simulink model "windModel"  (R2021a)
settings: Solver=VariableStepAuto  StartTime=0.0  StopTime=inf  RelTol=1e-3
undefined symbols (not defined in the file or in its folder): aircraft, FandM, MAV, plotprob
libraries: simulink x4
settings Model: Creator=DELL  LastModifiedBy=DELL

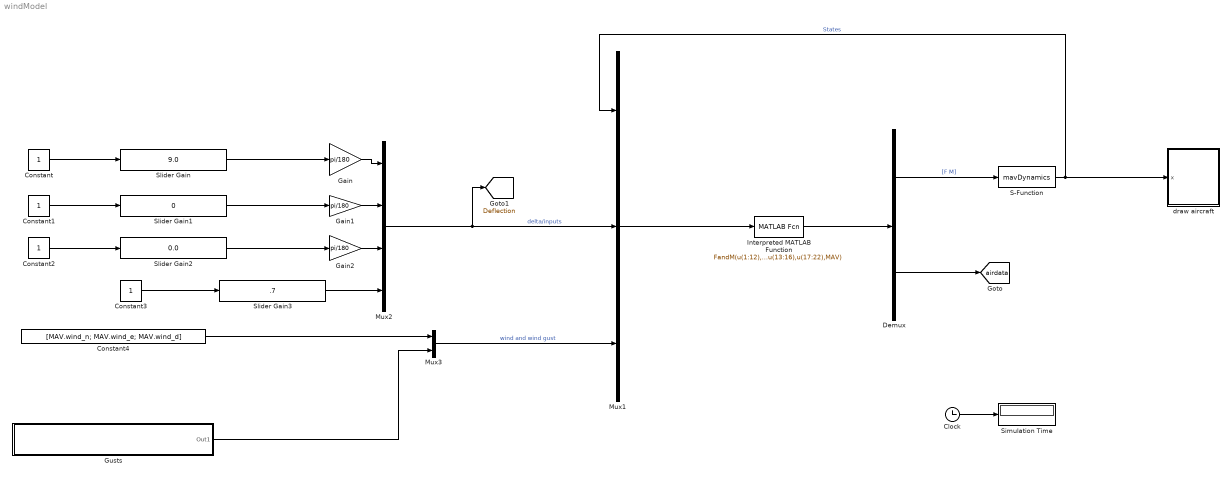
== system windModel ==
  Clock : Clock
  Constant{,1..3} (4 alike) : Constant
  Constant4 : Constant  Value=[MAV.wind_n; MAV.wind_e; MAV.wind_d]
  Demux : Demux  Outputs=[6;6]
  Gain : Gain  Gain=pi/180
  Gain1 : Gain  Gain=pi/180
  Gain2 : Gain  Gain=pi/180
  Gusts : Subsystem
  Interpreted MATLAB Function : MATLABFcn  MATLABFcn=FandM(u(1:12),u(13:16),u(17:22),MAV)  OutputDimensions=12
  Mux1 : Mux  Inputs=3
  Mux2 : Mux
  Mux3 : Mux  Inputs=2
  S-Function : S-Function  FunctionName=mavDynamics  Parameters=MAV  SFunctionDeploymentMode=off  EnableBusSupport=off
  Simulation Time : Display
  Slider Gain : simulink/Math Operations/Slider Gain  gain=9.0  low=-45  high=45
  Slider Gain1 : simulink/Math Operations/Slider Gain  gain=0  low=-45  high=45
  Slider Gain2 : simulink/Math Operations/Slider Gain  gain=0.0  low=-45  high=45
  Slider Gain3 : simulink/Math Operations/Slider Gain  gain=.7  low=0  high=1
  draw aircraft : Subsystem
  tag scope: Deflection=global, airdata=global
  wires:
  Constant/1 -> Slider Gain/1
  Constant3/1 -> Slider Gain3/1
  Slider Gain3/1 -> Mux2/4
  Mux2/1 -> [Deflection], Mux1/2  "delta/inputs"
  Mux1/1 -> Interpreted MATLAB Function/1
  Demux/1 -> S-Function/1  "[F M]"
  S-Function/1 -> Mux1/1, draw aircraft/1(x)  "States"
  Interpreted MATLAB Function/1 -> Demux/1
  Clock/1 -> Simulation Time/1
  Slider Gain/1 -> Gain/1
  Gain/1 -> Mux2/1
  Gain1/1 -> Mux2/2
  Slider Gain1/1 -> Gain1/1
  Constant1/1 -> Slider Gain1/1
  Gain2/1 -> Mux2/3
  Slider Gain2/1 -> Gain2/1
  Constant2/1 -> Slider Gain2/1
  Constant4/1 -> Mux3/1
  Mux3/1 -> Mux1/3  "wind and wind gust"
  Demux/2 -> [airdata]
  Gusts/1(Out1) -> Mux3/2

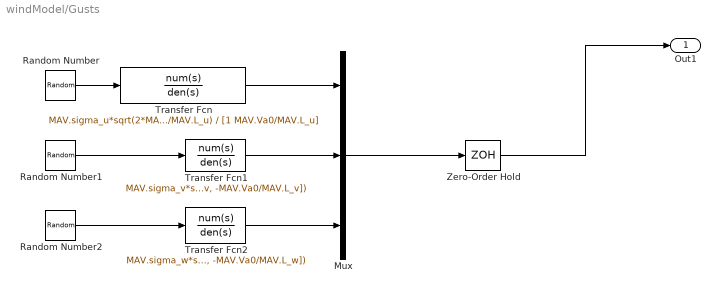
== system windModel/Gusts ==
  Mux : Mux  Inputs=3
  Random Number : RandomNumber  SampleTime=0.1
  Random Number1 : RandomNumber  SampleTime=0.1
  Random Number2 : RandomNumber  SampleTime=0.1
  Transfer Fcn : TransferFcn  Numerator=MAV.sigma_u*sqrt(2*MAV.Va0/MAV.L_u)  Denominator=[1 MAV.Va0/MAV.L_u]
  Transfer Fcn1 : TransferFcn  Numerator=MAV.sigma_v*sqrt(3*MAV.Va0/MAV.L_u)*[0, 1, MAV.Va0/sqrt(3)/MAV.L_v]  Denominator=poly([-MAV.Va0/MAV.L_v, -MAV.Va0/MAV.L_v])
  Transfer Fcn2 : TransferFcn  Numerator=MAV.sigma_w*sqrt(3*MAV.Va0/MAV.L_u)*[0, 1, MAV.Va0/sqrt(3)/MAV.L_w]  Denominator=poly([-MAV.Va0/MAV.L_w, -MAV.Va0/MAV.L_w])
  Zero-Order Hold : ZeroOrderHold  SampleTime=-1
  Out1 : Outport
  wires:
  Mux/1 -> Zero-Order Hold/1
  Random Number2/1 -> Transfer Fcn2/1
  Transfer Fcn1/1 -> Mux/2
  Random Number/1 -> Transfer Fcn/1
  Transfer Fcn/1 -> Mux/1
  Random Number1/1 -> Transfer Fcn1/1
  Transfer Fcn2/1 -> Mux/3
  Zero-Order Hold/1 -> Out1/1

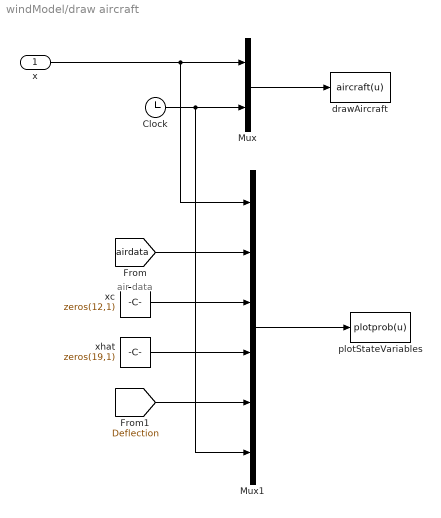
== system windModel/draw aircraft ==
  note: air data
  x : Inport
  Clock : Clock
  Mux : Mux  Inputs=2
  Mux1 : Mux  Inputs=6
  drawAircraft : MATLABFcn  MATLABFcn=aircraft(u)  OutputDimensions=0  SampleTime=0.1
  plotStateVariables : MATLABFcn  MATLABFcn=plotprob(u)  OutputDimensions=0  SampleTime=0.1
  xc : Constant  Value=zeros(12,1)
  xhat : Constant  Value=zeros(19,1)
  wires:
  Mux/1 -> drawAircraft/1
  x/1 -> Mux/1, Mux1/1
  Clock/1 -> Mux/2, Mux1/6
  Mux1/1 -> plotStateVariables/1
  xhat/1 -> Mux1/4
  xc/1 -> Mux1/3
  [Deflection] -> Mux1/5
  [airdata] -> Mux1/2
